simulink model "AM_DiffModulationIndex"  (R2021a)
settings: Solver=VariableStepAuto  StartTime=0.0  StopTime=1  RelTol=1e-3
libraries: dspfdesign x6
settings Model: Creator=ZephyrY  LastModifiedBy=ZephyrY

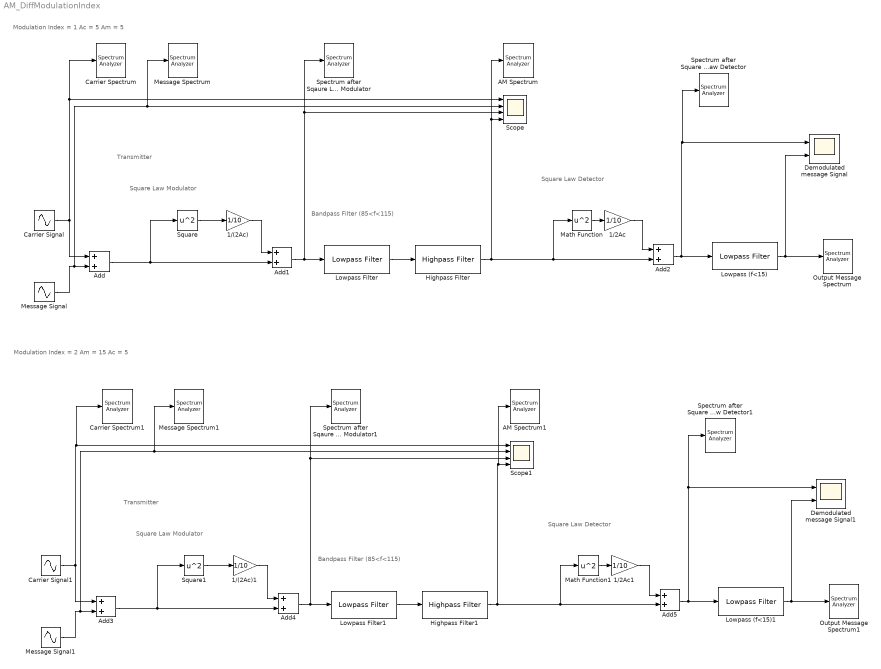
== system AM_DiffModulationIndex ==
  note: Modulation Index = 2
      | Am = 15
      | Ac = 5
  note: Modulation Index = 1
      | Ac = 5
      | Am = 5
  note: Square Law Detector
  note: Bandpass Filter (85<f<115)
  note: Square Law Modulator
  note: Transmitter
  note: Square Law Detector
  note: Bandpass Filter (85<f<115)
  note: Square Law Modulator
  note: Transmitter
  1/(2Ac) : Gain  Gain=1/10
  1/(2Ac)1 : Gain  Gain=1/10
  1/2Ac : Gain  Gain=1/10
  1/2Ac1 : Gain  Gain=1/10
  AM Spectrum : SpectrumAnalyzer
  AM Spectrum1 : SpectrumAnalyzer
  Add{,1..5} (6 alike) : Sum
  Carrier Signal : Sin  Amplitude=5  Frequency=2*pi*100  Phase=pi/2  SampleTime=1e-3
  Carrier Signal1 : Sin  Amplitude=5  Frequency=2*pi*100  Phase=pi/2  SampleTime=1e-3
  Carrier Spectrum : SpectrumAnalyzer
  Carrier Spectrum1 : SpectrumAnalyzer
  Demodulated message Signal : Scope  NumInputPorts=2
  Demodulated message Signal1 : Scope  NumInputPorts=2
  Highpass Filter : dspfdesign/Highpass Filter  FilterType=FIR  DesignForMinimumOrder=off  FilterOrder=50  StopbandFrequency=8e3  PassbandFrequency=85  StopbandAttenuation=80  PassbandRipple=0.1  InheritSampleRate=on  SampleRate=44100  SimulateUsing=Interpreted execution  roundingMode=Floor  coeffsDataTypeStr=fixdt(1,16)
  Highpass Filter1 : dspfdesign/Highpass Filter  FilterType=FIR  DesignForMinimumOrder=off  FilterOrder=50  StopbandFrequency=8e3  PassbandFrequency=85  StopbandAttenuation=80  PassbandRipple=0.1  InheritSampleRate=on  SampleRate=44100  SimulateUsing=Interpreted execution  roundingMode=Floor  coeffsDataTypeStr=fixdt(1,16)
  Lowpass (f<15) : dspfdesign/Lowpass Filter  FilterType=FIR  DesignForMinimumOrder=off  FilterOrder=200  PassbandFrequency=11  StopbandFrequency=12e3  PassbandRipple=0.1  StopbandAttenuation=80  InheritSampleRate=on  SampleRate=44100  SimulateUsing=Interpreted execution  roundingMode=Floor  coeffsDataTypeStr=fixdt(1,16)
  Lowpass (f<15)1 : dspfdesign/Lowpass Filter  FilterType=FIR  DesignForMinimumOrder=off  FilterOrder=200  PassbandFrequency=11  StopbandFrequency=12e3  PassbandRipple=0.1  StopbandAttenuation=80  InheritSampleRate=on  SampleRate=44100  SimulateUsing=Interpreted execution  roundingMode=Floor  coeffsDataTypeStr=fixdt(1,16)
  Lowpass Filter : dspfdesign/Lowpass Filter  FilterType=FIR  DesignForMinimumOrder=off  FilterOrder=50  PassbandFrequency=115  StopbandFrequency=12e3  PassbandRipple=0.1  StopbandAttenuation=80  InheritSampleRate=on  SampleRate=44100  SimulateUsing=Interpreted execution  roundingMode=Floor  coeffsDataTypeStr=fixdt(1,16)
  Lowpass Filter1 : dspfdesign/Lowpass Filter  FilterType=FIR  DesignForMinimumOrder=off  FilterOrder=50  PassbandFrequency=115  StopbandFrequency=12e3  PassbandRipple=0.1  StopbandAttenuation=80  InheritSampleRate=on  SampleRate=44100  SimulateUsing=Interpreted execution  roundingMode=Floor  coeffsDataTypeStr=fixdt(1,16)
  Math Function : Math  Operator=square  SaturateOnIntegerOverflow=on
  Math Function1 : Math  Operator=square  SaturateOnIntegerOverflow=on
  Message Signal : Sin  Amplitude=5  Frequency=2*pi*10  Phase=pi/2  SampleTime=1e-3
  Message Signal1 : Sin  Amplitude=15  Frequency=2*pi*10  Phase=pi/2  SampleTime=1e-3
  Message Spectrum : SpectrumAnalyzer
  Message Spectrum1 : SpectrumAnalyzer
  Output Message Spectrum : SpectrumAnalyzer
  Output Message Spectrum1 : SpectrumAnalyzer
  Scope : Scope  NumInputPorts=4
  Scope1 : Scope  NumInputPorts=4
  Spectrum after Square Law Detector : SpectrumAnalyzer
  Spectrum after Square Law Detector1 : SpectrumAnalyzer
  Spectrum after Sqaure Law Modulator : SpectrumAnalyzer
  Spectrum after Sqaure Law Modulator1 : SpectrumAnalyzer
  Square : Math  Operator=square  SaturateOnIntegerOverflow=on
  Square1 : Math  Operator=square  SaturateOnIntegerOverflow=on
  wires:
  Add/1 -> Add1/2, Square/1
  Square/1 -> 1/(2Ac)/1
  Math Function/1 -> 1/2Ac/1
  Add1/1 -> Spectrum after Sqaure Law Modulator/1, Scope/3, Lowpass Filter/1
  Lowpass (f<15)/1 -> Output Message Spectrum/1, Demodulated message Signal/2
  Highpass Filter/1 -> AM Spectrum/1, Scope/4, Add2/2, Math Function/1
  Lowpass Filter/1 -> Highpass Filter/1
  1/2Ac/1 -> Add2/1
  Message Signal/1 -> Message Spectrum/1, Scope/2, Add/2
  Carrier Signal/1 -> Add/1, Carrier Spectrum/1, Scope/1
  Add2/1 -> Spectrum after Square Law Detector/1, Demodulated message Signal/1, Lowpass (f<15)/1
  1/(2Ac)/1 -> Add1/1
  Add3/1 -> Add4/2, Square1/1
  Square1/1 -> 1/(2Ac)1/1
  Math Function1/1 -> 1/2Ac1/1
  Add4/1 -> Spectrum after Sqaure Law Modulator1/1, Scope1/3, Lowpass Filter1/1
  Lowpass (f<15)1/1 -> Output Message Spectrum1/1, Demodulated message Signal1/2
  Highpass Filter1/1 -> AM Spectrum1/1, Scope1/4, Add5/2, Math Function1/1
  Lowpass Filter1/1 -> Highpass Filter1/1
  1/2Ac1/1 -> Add5/1
  Message Signal1/1 -> Message Spectrum1/1, Scope1/2, Add3/2
  Carrier Signal1/1 -> Add3/1, Carrier Spectrum1/1, Scope1/1
  Add5/1 -> Spectrum after Square Law Detector1/1, Demodulated message Signal1/1, Lowpass (f<15)1/1
  1/(2Ac)1/1 -> Add4/1
